simulink model "sampleModel1682"  (R2023a)
settings: Solver=VariableStepAuto  StartTime=0.0  StopTime=10.0  RelTol=1e-3
libraries: hdlsllib x7, simulink x3
settings Model: Creator=user1  LastModifiedBy=user1

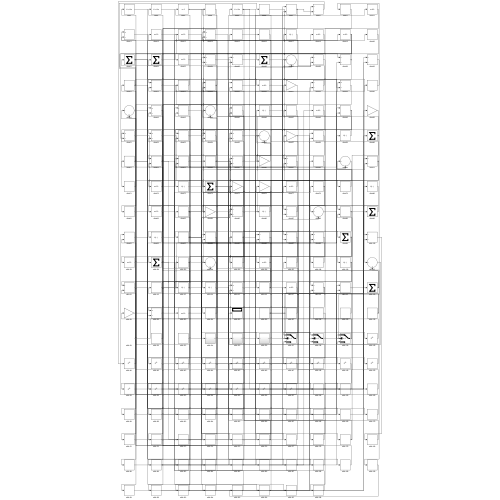
[thumbnail: Simulink's stored preview of the top-level diagram]
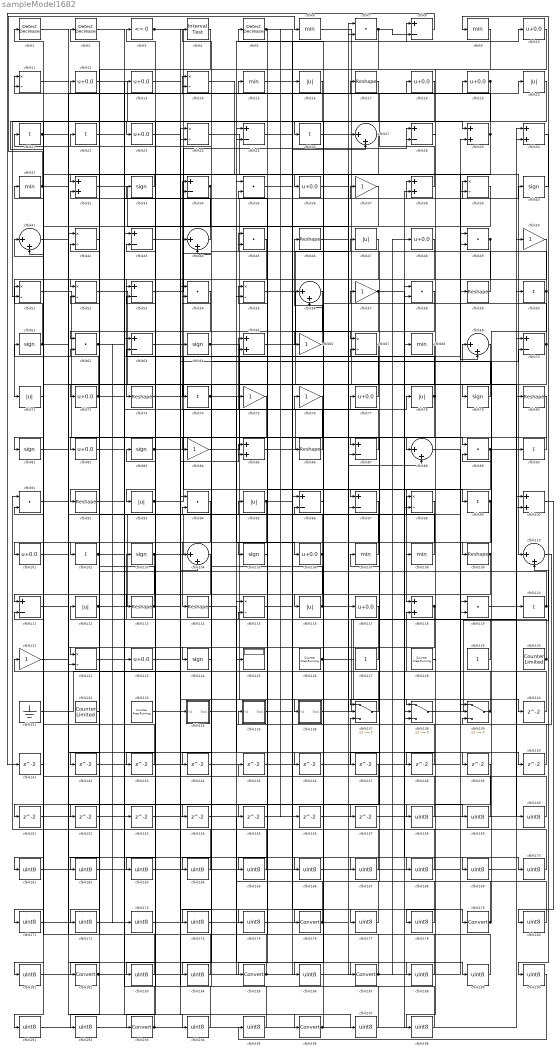
== system sampleModel1682 ==
  cfblk1 : simulink/Logic and Bit Operations/Detect Decrease  vinit=0.0  OutDataTypeStr=boolean
      settings: LibrarySourceBlock=|
      | hdlsllib/Logic and Bit
      | Operations/Detect
      | Decrease
  cfblk{10,12..13,18..19,23,36,48,72,77,82,101,106,117,123} (15 alike) : Bias  Bias=0.0  SaturateOnIntegerOverflow=off
  cfblk{29..30,32,38,65,85,100,118} (8 alike) : Sum
  cfblk{21..22,26,60,74,90,99,102,120} (9 alike) : Sum  Inputs=+
  cfblk{33,40,61,64,79,81,83,103,105,124} (10 alike) : Signum
  cfblk{27,41,44,56,69,88,104,110} (8 alike) : Sum  Inputs=|++
  cfblk{6,9,15,31,68,107..108} (7 alike) : MinMax
  cfblk{17,46,59,73,80,86,92,109,113..114} (10 alike) : Reshape
  cfblk{11,14,24,39,42,51..52,55,67,98,115,122} (12 alike) : Product  Inputs=*/  RndMeth=Zero  SaturateOnIntegerOverflow=on
  cfblk{8,25,28,34,43,53,63,70,87,96..97,111} (12 alike) : Sum  Inputs=+-
  cfblk{16,20,47,71,78,93,95,112,116} (9 alike) : Abs  SaturateOnIntegerOverflow=off
  cfblk{7,35,45,49,54,58,62,89,91,94,119} (11 alike) : DotProduct  OutDataTypeStr=Inherit: Inherit via internal rule
  cfblk{37,50,57,66,75..76,84,121} (8 alike) : Gain
  cfblk125 : Display
  cfblk126 : hdlsllib/Sources/Counter Free-Running  NumBits=16  tsamp=-1
  cfblk127 : Constant  SampleTime=-1
  cfblk128 : hdlsllib/Sources/Counter Free-Running  NumBits=16  tsamp=-1
  cfblk129 : Constant  SampleTime=-1
  cfblk130 : hdlsllib/Sources/Counter Limited  uplimit=7  tsamp=-1
  cfblk131 : Ground
  cfblk132 : hdlsllib/Sources/Counter Limited  uplimit=7  tsamp=-1
  cfblk133 : hdlsllib/Sources/Counter Free-Running  NumBits=16  tsamp=-1
  cfblk134 : Subsystem
      settings: LibrarySourceBlock=|
      | hdlsllib/Ports &
      | Subsystems/Subsystem
  cfblk135 : Subsystem
      settings: LibrarySourceBlock=|
      | hdlsllib/Ports &
      | Subsystems/Subsystem
  cfblk136 : Subsystem
      settings: LibrarySourceBlock=|
      | hdlsllib/Ports &
      | Subsystems/Subsystem
  cfblk137 : Switch  SaturateOnIntegerOverflow=off  InputSameDT=off
  cfblk138 : Switch  SaturateOnIntegerOverflow=off  InputSameDT=off
  cfblk139 : Switch  SaturateOnIntegerOverflow=off  InputSameDT=off
  cfblk{140..157} (18 alike) : Delay  SampleTime=1
  cfblk{158..175,177..178,180..181,183..184,186,188..192,194..195,197..198} (34 alike) : DataTypeConversion  OutDataTypeStr=uint8  SaturateOnIntegerOverflow=off  RndMeth=Floor
  cfblk{176,179,182,185,187,193,196} (7 alike) : DataTypeConversion  SaturateOnIntegerOverflow=off  RndMeth=Floor
  cfblk2 : simulink/Logic and Bit Operations/Detect Decrease  vinit=0.0  OutDataTypeStr=boolean
      settings: LibrarySourceBlock=|
      | hdlsllib/Logic and Bit
      | Operations/Detect
      | Decrease
  cfblk3 : hdlsllib/Logic and Bit Operations/Compare To Zero  relop=<=  OutDataTypeStr=boolean
  cfblk4 : hdlsllib/Logic and Bit Operations/Interval Test  IntervalClosedRight=on  uplimit=0.5  IntervalClosedLeft=on  lowlimit=-0.5  OutDataTypeStr=boolean
  cfblk5 : simulink/Logic and Bit Operations/Detect Decrease  vinit=0.0  OutDataTypeStr=boolean
      settings: LibrarySourceBlock=|
      | hdlsllib/Logic and Bit
      | Operations/Detect
      | Decrease
  wires:
  cfblk116/1 -> cfblk15/1, cfblk63/2, cfblk138/1
  cfblk6/1 -> cfblk79/1
  cfblk64/1 -> cfblk97/1, cfblk98/2
  cfblk59/1 -> cfblk21/1
  cfblk84/1 -> cfblk37/1
  cfblk70/1 -> cfblk5/1, cfblk154/1, cfblk186/1
  cfblk85/1 -> cfblk7/1
  cfblk93/1 -> cfblk77/1, cfblk85/1, cfblk85/2
  cfblk26/1 -> cfblk110/1
  cfblk14/1 -> cfblk36/1
  cfblk48/1 -> cfblk73/1
  cfblk18/1 -> cfblk93/1
  cfblk38/1 -> cfblk11/1
  cfblk12/1 -> cfblk29/1
  cfblk107/1 -> cfblk83/1
  cfblk20/1 -> cfblk26/1
  cfblk126/1 -> cfblk50/1, cfblk139/2
  cfblk66/1 -> cfblk46/1
  cfblk74/1 -> cfblk136/1(In1), cfblk106/1
  cfblk71/1 -> cfblk23/1
  cfblk3/1 -> cfblk118/1, cfblk87/1
  cfblk127/1 -> cfblk122/1
  cfblk95/1 -> cfblk114/1, cfblk99/1
  cfblk136/1(Out1) -> cfblk90/1
  cfblk63/1 -> cfblk134/1(In1)
  cfblk45/1 -> cfblk52/1
  cfblk113/1 -> cfblk12/1, cfblk138/3
  cfblk33/1 -> cfblk32/1
  cfblk44/1 -> cfblk22/1
  cfblk50/1 -> cfblk71/1
  cfblk34/1 -> cfblk102/1, cfblk14/2
  cfblk42/1 -> cfblk182/1
  cfblk106/1 -> cfblk2/1, cfblk191/1
  cfblk89/1 -> cfblk120/1, cfblk165/1
  cfblk10/1 -> cfblk82/1
  cfblk60/1 -> cfblk109/1, cfblk33/1
  cfblk22/1 -> cfblk18/1
  cfblk43/1 -> cfblk196/1
  cfblk122/1 -> cfblk13/1
  cfblk108/1 -> cfblk3/1
  cfblk49/1 -> cfblk116/1, cfblk53/1
  cfblk92/1 -> cfblk19/1
  cfblk7/1 -> cfblk92/1, cfblk8/2
  cfblk109/1 -> cfblk157/1, cfblk192/1
  cfblk27/1 -> cfblk97/2
  cfblk138/1 -> cfblk110/2
  cfblk16/1 -> cfblk101/1
  cfblk115/1 -> cfblk38/1
  cfblk51/1 -> cfblk123/1
  cfblk65/1 -> cfblk27/1
  cfblk110/1 -> cfblk135/1(In1)
  cfblk52/1 -> cfblk86/1
  cfblk55/1 -> cfblk100/1
  cfblk41/1 -> cfblk187/1
  cfblk39/1 -> cfblk81/1
  cfblk134/1(Out1) -> cfblk8/1
  cfblk29/1 -> cfblk111/1, cfblk17/1
  cfblk112/1 -> cfblk49/1, cfblk67/2
  cfblk53/1 -> cfblk28/1
  cfblk24/1 -> cfblk69/2
  cfblk130/1 -> cfblk103/1, cfblk44/1
  cfblk47/1 -> cfblk113/1
  cfblk133/1 -> cfblk98/1
  cfblk124/1 -> cfblk4/1
  cfblk103/1 -> cfblk49/2, cfblk172/1
  cfblk82/1 -> cfblk78/1
  cfblk131/1 -> cfblk24/1
  cfblk80/1 -> cfblk137/1
  cfblk137/1 -> cfblk31/1
  cfblk19/1 -> cfblk66/1, cfblk51/2, cfblk152/1
  cfblk25/1 -> cfblk179/1
  cfblk40/1 -> cfblk9/1
  cfblk90/1 -> cfblk88/1
  cfblk15/1 -> cfblk10/1
  cfblk87/1 -> cfblk65/1
  cfblk31/1 -> cfblk6/1, cfblk74/1
  cfblk36/1 -> cfblk88/2
  cfblk129/1 -> cfblk32/2
  cfblk37/1 -> cfblk72/1
  cfblk120/1 -> cfblk45/1, cfblk62/2
  cfblk86/1 -> cfblk34/1
  cfblk61/1 -> cfblk20/1, cfblk51/1, cfblk168/1
  cfblk132/1 -> cfblk52/2
  cfblk23/1 -> cfblk64/1
  cfblk73/1 -> cfblk40/1
  cfblk72/1 -> cfblk61/1, cfblk39/1
  cfblk96/1 -> cfblk176/1
  cfblk46/1 -> cfblk28/2
  cfblk139/1 -> cfblk107/1, cfblk44/2
  cfblk57/1 -> cfblk87/2, cfblk170/1
  cfblk62/1 -> cfblk65/2, cfblk153/1
  cfblk77/1 -> cfblk34/2
  cfblk118/1 -> cfblk115/2, cfblk122/2
  cfblk21/1 -> cfblk89/1, cfblk39/2
  cfblk9/1 -> cfblk108/1
  cfblk17/1 -> cfblk24/2
  cfblk32/1 -> cfblk137/2
  cfblk105/1 -> cfblk55/1
  cfblk83/1 -> cfblk75/1, cfblk70/2, cfblk183/1
  cfblk101/1 -> cfblk95/1
  cfblk99/1 -> cfblk151/1, cfblk184/1
  cfblk75/1 -> cfblk124/1
  cfblk79/1 -> cfblk14/1
  cfblk5/1 -> cfblk67/1, cfblk155/1, cfblk156/1
  cfblk58/1 -> cfblk105/1
  cfblk54/1 -> cfblk193/1
  cfblk78/1 -> cfblk84/1, cfblk53/2, cfblk147/1
  cfblk102/1 -> cfblk149/1, cfblk173/1
  cfblk68/1 -> cfblk185/1
  cfblk56/1 -> cfblk62/1
  cfblk35/1 -> cfblk27/2
  cfblk88/1 -> cfblk140/1
  cfblk140/1 -> cfblk118/2
  cfblk8/1 -> cfblk141/1
  cfblk141/1 -> cfblk11/2
  cfblk76/1 -> cfblk142/1
  cfblk142/1 -> cfblk137/3
  cfblk97/1 -> cfblk143/1
  cfblk143/1 -> cfblk111/2
  cfblk69/1 -> cfblk144/1
  cfblk144/1 -> cfblk38/2
  cfblk81/1 -> cfblk146/1
  cfblk146/1 -> cfblk29/2
  cfblk28/1 -> cfblk148/1
  cfblk148/1 -> cfblk115/1
  cfblk114/1 -> cfblk150/1
  cfblk150/1 -> cfblk89/2
  cfblk151/1 -> cfblk55/2
  cfblk152/1 -> cfblk58/2
  cfblk153/1 -> cfblk70/1
  cfblk155/1 -> cfblk139/1
  cfblk156/1 -> cfblk100/2
  cfblk157/1 -> cfblk60/1
  cfblk1/1 -> cfblk158/1
  cfblk158/1 -> cfblk47/1
  cfblk145/1 -> cfblk159/1
  cfblk159/1 -> cfblk1/1
  cfblk119/1 -> cfblk160/1
  cfblk160/1 -> cfblk69/1
  cfblk67/1 -> cfblk161/1
  cfblk161/1 -> cfblk119/1
  cfblk4/1 -> cfblk162/1
  cfblk162/1 -> cfblk119/2
  cfblk94/1 -> cfblk163/1
  cfblk163/1 -> cfblk125/1
  cfblk98/1 -> cfblk164/1
  cfblk164/1 -> cfblk94/1
  cfblk165/1 -> cfblk94/2
  cfblk91/1 -> cfblk166/1
  cfblk166/1 -> cfblk76/1
  cfblk135/1(Out1) -> cfblk167/1
  cfblk167/1 -> cfblk91/1
  cfblk168/1 -> cfblk91/2
  cfblk121/1 -> cfblk169/1
  cfblk169/1 -> cfblk80/1
  cfblk170/1 -> cfblk121/1
  cfblk104/1 -> cfblk171/1
  cfblk171/1 -> cfblk16/1
  cfblk172/1 -> cfblk104/1
  cfblk173/1 -> cfblk104/2
  cfblk117/1 -> cfblk174/1
  cfblk174/1 -> cfblk35/1
  cfblk13/1 -> cfblk175/1
  cfblk175/1 -> cfblk117/1
  cfblk176/1 -> cfblk145/1, cfblk35/2
  cfblk123/1 -> cfblk177/1
  cfblk177/1 -> cfblk96/1
  cfblk128/1 -> cfblk178/1
  cfblk178/1 -> cfblk96/2
  cfblk179/1 -> cfblk139/3, cfblk57/1
  cfblk100/1 -> cfblk180/1
  cfblk180/1 -> cfblk25/1
  cfblk147/1 -> cfblk181/1
  cfblk181/1 -> cfblk25/2
  cfblk182/1 -> cfblk56/1, cfblk7/2
  cfblk183/1 -> cfblk42/1
  cfblk184/1 -> cfblk42/2
  cfblk185/1 -> cfblk59/1, cfblk112/1
  cfblk186/1 -> cfblk68/1
  cfblk187/1 -> cfblk45/2, cfblk48/1
  cfblk111/1 -> cfblk188/1
  cfblk188/1 -> cfblk41/1
  cfblk154/1 -> cfblk189/1
  cfblk189/1 -> cfblk41/2
  cfblk30/1 -> cfblk190/1
  cfblk191/1 -> cfblk30/1
  cfblk192/1 -> cfblk30/2
  cfblk193/1 -> cfblk138/2, cfblk63/1
  cfblk2/1 -> cfblk194/1
  cfblk194/1 -> cfblk54/1
  cfblk190/1 -> cfblk195/1
  cfblk195/1 -> cfblk54/2
  cfblk196/1 -> cfblk56/2, cfblk58/1
  cfblk11/1 -> cfblk197/1
  cfblk197/1 -> cfblk43/1
  cfblk149/1 -> cfblk198/1
  cfblk198/1 -> cfblk43/2

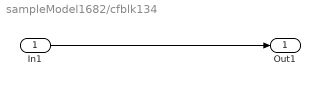
== system sampleModel1682/cfblk134 ==
  In1 : Inport
  Out1 : Outport
  wires:
  In1/1 -> Out1/1

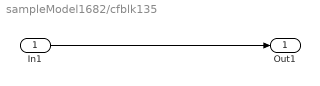
== system sampleModel1682/cfblk135 ==
  In1 : Inport
  Out1 : Outport
  wires:
  In1/1 -> Out1/1

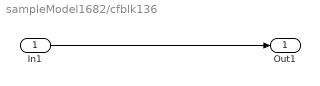
== system sampleModel1682/cfblk136 ==
  In1 : Inport
  Out1 : Outport
  wires:
  In1/1 -> Out1/1
